simulink model "VerificationSubsystem"  (R2021b)
settings: Solver=FixedStepDiscrete  StartTime=0.0  StopTime=10.0  FixedStep=0.2  RelTol=1e-3
undefined symbols (not defined in the file or in its folder): sldvsubsys
libraries: simulink x2, sldvlib x1
settings Model: DVExtractedSubsystem=Verification Subsystem  Creator=Alessandro  LastModifiedBy=Alessandro
settings DebuggingCC: FrameProcessingCompatibilityMsg=none
settings ConfigComp: DVMode=PropertyProving  DVTestSuiteOptimization=Auto  DVDetectOutOfBounds=on  DVModelReferenceHarness=on

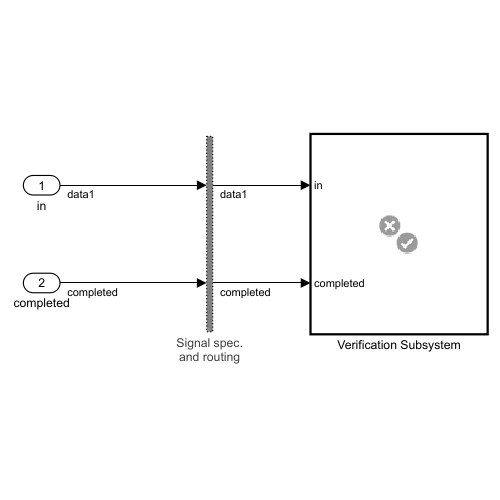
[thumbnail: Simulink's stored preview of the top-level diagram]
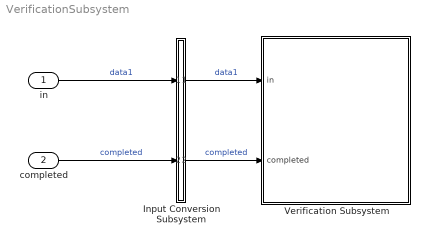
== system VerificationSubsystem ==
  in : Inport  OutDataTypeStr=double  PortDimensions=[1]  SampleTime=0.2  Interpolate=off
  completed : Inport  Port=2  OutDataTypeStr=double  PortDimensions=[1]  SampleTime=0.2  Interpolate=off
  Input Conversion Subsystem : Subsystem  Tag=__SLT_ICS__  Description=|
      | Signal spec.
      | and routing
      settings: AttributesFormatString=%<Description>
  Verification Subsystem : Subsystem  Tag=VerificationSubsystem  DisableCoverage=on  LoadFcn=sldvsubsys('check')  TreatAsAtomicUnit=on  SimViewingDevice=on  mask(VerificationSubsystem){}
      mask init:
      | sldvsubsys('maskInit');
      settings: CopyFcn=sldvsubsys('copy');  OpenFcn=open_system(gcb,'force');
      settings: PreSaveFcn=|
      | set_param(gcb,'SimViewingDevice','on');
      | sldvsubsys('check');
      mask Help: helpview(fullfile(docroot,'toolbox','sldv','sldv.map'),'verificationsubsystem')
      mask Display: image(imread('sldvicon_versubsys.png','BackGroundColor',[1 1 1]),'center');
  wires:
  in/1 -> Input Conversion Subsystem/1(Inport_1)  "data1"
  completed/1 -> Input Conversion Subsystem/2(Inport_2)  "completed"
  Input Conversion Subsystem/1(Outport_1) -> Verification Subsystem/1(in)  "data1"
  Input Conversion Subsystem/2(Outport_2) -> Verification Subsystem/2(completed)  "completed"

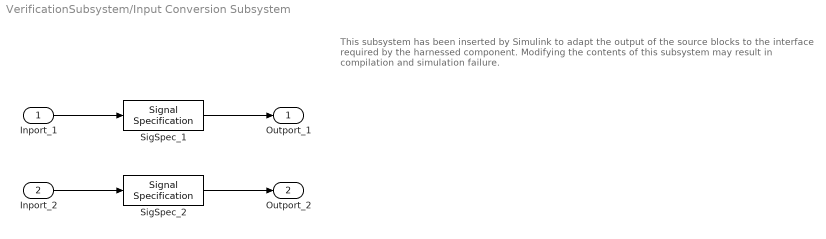
== system VerificationSubsystem/Input Conversion Subsystem ==
  note: This subsystem has been inserted by Simulink to adapt the output of the source blocks to the interface required by the harnessed component.
      |  Modifying the contents of this subsystem may result in compilation and simulation failure.
  Inport_1 : Inport
  Inport_2 : Inport  Port=2
  SigSpec_1 : SignalSpecification  OutDataTypeStr=double  Dimensions=[1]  SampleTime=0.2
  SigSpec_2 : SignalSpecification  OutDataTypeStr=double  Dimensions=[1]  SampleTime=0.2
  Outport_1 : Outport
  Outport_2 : Outport  Port=2
  wires:
  SigSpec_1/1 -> Outport_1/1
  Inport_1/1 -> SigSpec_1/1
  SigSpec_2/1 -> Outport_2/1
  Inport_2/1 -> SigSpec_2/1

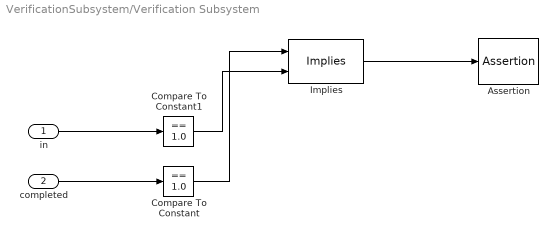
== system VerificationSubsystem/Verification Subsystem ==
  in : Inport
  completed : Inport  Port=2
  Assertion : Assertion  StopWhenAssertionFail=off
  Compare To Constant : simulink/Logic and Bit Operations/Compare To Constant  relop===  const=1.0  OutDataTypeStr=boolean
  Compare To Constant1 : simulink/Logic and Bit Operations/Compare To Constant  relop===  const=1.0  OutDataTypeStr=boolean
  Implies : sldvlib/Verification Utilities/Implies
      settings: SourceProductBaseCode=SL
  wires:
  Implies/1 -> Assertion/1
  Compare To Constant1/1 -> Implies/2
  Compare To Constant/1 -> Implies/1
  in/1 -> Compare To Constant1/1
  completed/1 -> Compare To Constant/1
